simulink model "BlinkLED"  (R2014a)
settings: Solver=FixedStepDiscrete  StartTime=0.0  StopTime=inf  FixedStep=0.005  RelTol=1e-3  SampleTimeConstraint=Specified
libraries: simulink x2
settings Model: Creator=ses  LastModifiedBy=ses
settings SolverCC: PositivePriorityOrder=on
settings OptimizationCC: OptimizeModelRefInitCode=on  LifeSpan=Inf  MaxStackSize=64
settings HardwareCC: ProdLargestAtomicInteger=Long  ProdLargestAtomicFloat=Double  ProdEndianess=LittleEndian  ProdHWDeviceType=ARM Compatible->ARM Cortex
settings RTWCC: SystemTargetFile=ert_linux.tlc  MakeCommand=make_rtw CC=arm-linux-gnueabihf-gcc  TemplateMakefile=ert_linux.tmf  Description=Linux Embedded Coder  ProcessScript=ert_linux_make_rtw_hook
settings CodeAppCC: IgnoreCustomStorageClasses=off
settings STFCustomTargetCC: ModelReferenceCompliant=off  ConcurrentExecutionCompliant=off  GeneratePreprocessorConditionals=Use local settings  CombineOutputUpdateFcns=on  ERTCustomFileBanners=on  SupportContinuousTime=off  MATLABClassNameForMDSCustomization=Simulink.SoftwareTarget.ERTCustomization  GRTInterface=off  SystemTargetFile=ert_linux.tlc
settings ERTTargetCC: GenerateSampleERTMain=off  ModelReferenceCompliant=off  SupportNonInlinedSFcns=on  ERTCustomFileTemplate=ert_linux_file_process.tlc

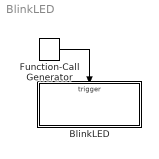
== system BlinkLED ==
  BlinkLED : Subsystem  TreatAsAtomicUnit=on
  Function-Call Generator : simulink/Ports & Subsystems/Function-Call Generator  sample_time=0.005  numberOfIterations=1
  wires:
  Function-Call Generator/1 -> BlinkLED/Trigger

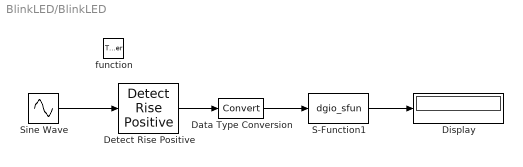
== system BlinkLED/BlinkLED ==
  function : TriggerPort  TriggerType=function-call  SampleTime=0.005
  Data Type Conversion : DataTypeConversion
  Detect Rise Positive : simulink/Logic and Bit Operations/Detect Rise Positive  vinit=0  InputProcessing=Inherited  OutDataTypeStr=boolean
  Display : Display
  S-Function1 : S-Function  FunctionName=dgio_sfun  EnableBusSupport=off
  Sine Wave : Sin  Frequency=2  Phase=-pi/8
  wires:
  Detect Rise Positive/1 -> Data Type Conversion/1
  S-Function1/1 -> Display/1
  Data Type Conversion/1 -> S-Function1/1
  Sine Wave/1 -> Detect Rise Positive/1
